simulink model "new_PV_array"  (Simulink 8.5)
settings: Solver=ode45  StartTime=0.0  StopTime=10  RelTol=1e-3
libraries: powerlib x1
settings Model: Creator=farhanm  LastModifiedBy=jiax
settings DebuggingCC: SolverPrmCheckMsg=warning  FcnCallInpInsideContextMsg=UseLocalSettings
settings ConfigurationSet: Description=SimMechanics 2G

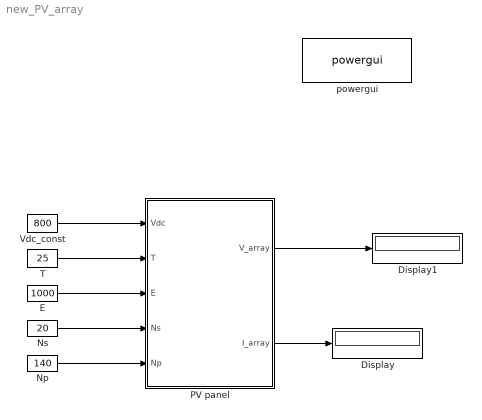
== system new_PV_array ==
  Display : Display
  Display1 : Display
  E : Constant  Value=1000
  Np : Constant  Value=140
  Ns : Constant  Value=20
  "PV panel " : Subsystem  mask{Voc=43.8, Isc=5, Vmpp=35, Impp=4.58, beta_Voc=-0.1, alpha_Isc=0.00002, Ncell=40}
      mask prompts: Voc "Open Circuit Voltage Voc (V)"; Isc "Short Circuit Current Isc (A)"; Vmpp "Voltage at Maximum Power Point Vmpp (V)"; Impp "Current at Maximum Power Point Impp (A)"; beta_Voc "Temperature Coefficient of Voc (%/deg.C)"; alpha_Isc "Temperature Coefficient of Isc (%/deg.C)"; Ncell "Cells per Module (Ncell)"
  T : Constant  Value=25
  Vdc_const : Constant  Value=800
  powergui : powerlib/powergui  Priority=1  SimulationMode=Discrete  SolverType=Tustin/Backward Euler (TBE)  SampleTime=50e-6  frequency=60  SPID=off  DisableSnubberDevices=off  DisableRonSwitches=off  DisableVfSwitches=off  SwTol=0  DisplayEquations=off  Interpol=off  methode=off  Ts=0  FunctionMessages=off  echomessages=off  HookPort=off  EnableUseOfTLC=off  x0status=blocks  frequencyindice=50  Pbase=100e6  ErrMax=1e-4  Iterations=50  UnitsV=kV  UnitsW=MW  buscounter=0  RestoreLinks=warning  ResistiveCurrentMeasurement=off  Frange=[0:2:500]  Ylog=off  Xlog=on  ShowGrid=off  save=off  variable=ZData  structure=0  ZoomFFT=off  StartTime=0.0  cycles=1  DisplayStyle=1  fundamental=60  FreqAxis=off  MaxFrequency=1000  frequencyindicesteady=1  RmsSteady=1  display=off
  wires:
  T/1 -> "PV panel "/2(T)
  E/1 -> "PV panel "/3(E)
  Np/1 -> "PV panel "/5(Np)
  Ns/1 -> "PV panel "/4(Ns)
  "PV panel "/1(V_array) -> Display1/1
  Vdc_const/1 -> "PV panel "/1(Vdc)
  "PV panel "/2(I_array) -> Display/1

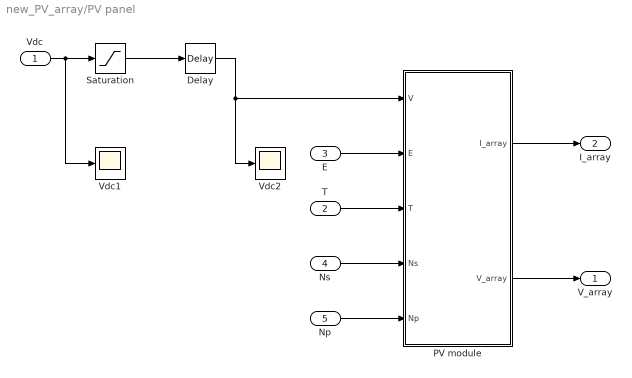
== system new_PV_array/PV panel  ==
  Vdc : Inport
  T : Inport  Port=2
  E : Inport  Port=3
  Ns : Inport  Port=4
  Np : Inport  Port=5
  Delay : TransportDelay  DelayTime=0.05
  PV module : Subsystem
  Saturation : Saturate  UpperLimit=876  LowerLimit=0
  Vdc1 : Scope
      settings: SaveName=ScopeData19
  Vdc2 : Scope
      settings: SaveName=ScopeData20
  V_array : Outport
  I_array : Outport  Port=2
  wires:
  Saturation/1 -> Delay/1
  E/1 -> PV module/2(E)
  T/1 -> PV module/3(T)
  Vdc/1 -> Saturation/1, Vdc1/1
  Delay/1 -> PV module/1(V), Vdc2/1
  Ns/1 -> PV module/4(Ns)
  Np/1 -> PV module/5(Np)
  PV module/1(I_array) -> I_array/1
  PV module/2(V_array) -> V_array/1

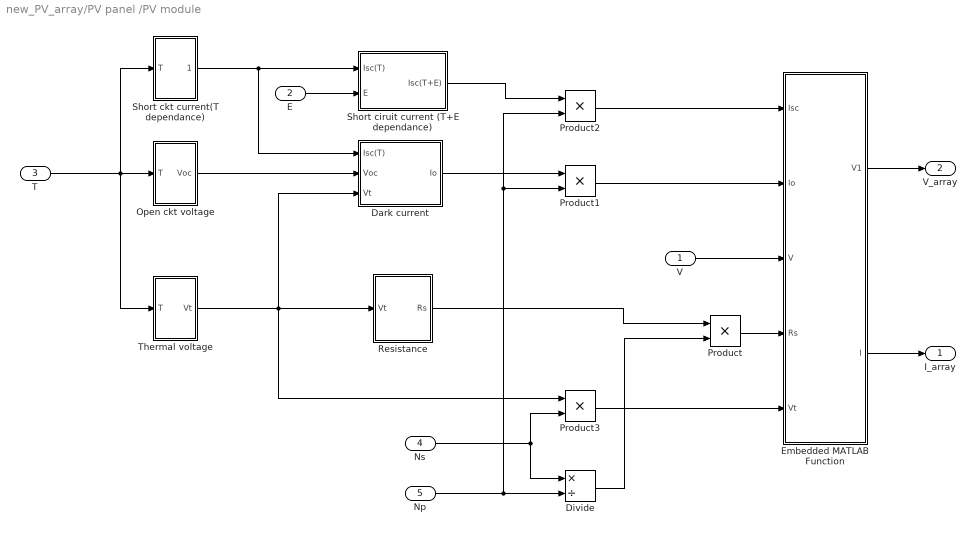
== system new_PV_array/PV panel /PV module ==
  V : Inport
  E : Inport  Port=2
  T : Inport  Port=3
  Ns : Inport  Port=4
  Np : Inport  Port=5
  Dark current : Subsystem
  Divide : Product  Inputs=*/
  Embedded MATLAB Function : MATLAB Function  TreatAsAtomicUnit=on
  Open ckt voltage : Subsystem
  Product{,1..3} (4 alike) : Product
  Resistance : Subsystem
  Short ciruit current (T+E dependance) : Subsystem
  "Short ckt current(T dependance) " : Subsystem
  Thermal voltage : Subsystem
  I_array : Outport
  V_array : Outport  Port=2
  wires:
  Thermal voltage/1(Vt) -> Product3/1, Resistance/1(Vt), Dark current/3(Vt)
  T/1 -> "Short ckt current(T dependance) "/1(T), Thermal voltage/1(T), Open ckt voltage/1(T)
  E/1 -> Short ciruit current (T+E dependance)/2(E)
  Open ckt voltage/1(Voc) -> Dark current/2(Voc)
  Embedded MATLAB Function/2(I) -> I_array/1
  Embedded MATLAB Function/1(V1) -> V_array/1
  V/1 -> Embedded MATLAB Function/3(V)
  Ns/1 -> Product3/2, Divide/1
  Np/1 -> Divide/2, Product1/2, Product2/2
  Product/1 -> Embedded MATLAB Function/4(Rs)
  Product1/1 -> Embedded MATLAB Function/2(Io)
  Product2/1 -> Embedded MATLAB Function/1(Isc)
  Product3/1 -> Embedded MATLAB Function/5(Vt)
  Dark current/1(Io) -> Product1/1
  Resistance/1(Rs) -> Product/1
  Divide/1 -> Product/2
  "Short ckt current(T dependance) "/1(Isc(T)) -> Dark current/1(Isc(T)), Short ciruit current (T+E dependance)/1(Isc(T))
  Short ciruit current (T+E dependance)/1(Isc(T+E)) -> Product2/1

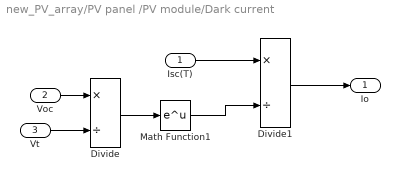
== system new_PV_array/PV panel /PV module/Dark current ==
  Isc(T) : Inport
  Voc : Inport  Port=2
  Vt : Inport  Port=3
  Divide : Product  Inputs=*/
  Divide1 : Product  Inputs=*/
  Math Function1 : Math  SaturateOnIntegerOverflow=on
  Io : Outport
  wires:
  Divide/1 -> Math Function1/1
  Math Function1/1 -> Divide1/2
  Vt/1 -> Divide/2
  Voc/1 -> Divide/1
  Isc(T)/1 -> Divide1/1
  Divide1/1 -> Io/1

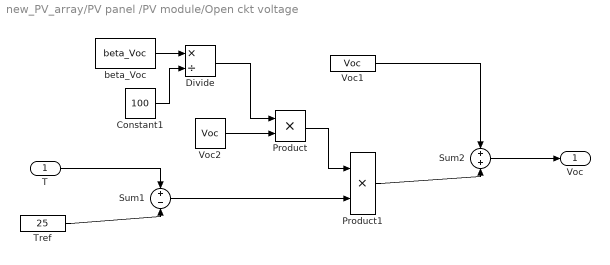
== system new_PV_array/PV panel /PV module/Open ckt voltage ==
  T : Inport
  Constant1 : Constant  Value=100
  Divide : Product  Inputs=*/
  Product : Product
  Product1 : Product  RndMeth=Zero
  Sum1 : Sum  Inputs=+-
  Sum2 : Sum
  Tref : Constant  Value=25
  Voc1 : Constant  Value=Voc
  Voc2 : Constant  Value=Voc
  beta_Voc : Constant  Value=beta_Voc
  Voc : Outport
  wires:
  Tref/1 -> Sum1/2
  T/1 -> Sum1/1
  Sum1/1 -> Product1/2
  Voc1/1 -> Sum2/1
  Product1/1 -> Sum2/2
  Sum2/1 -> Voc/1
  beta_Voc/1 -> Divide/1
  Constant1/1 -> Divide/2
  Divide/1 -> Product/1
  Voc2/1 -> Product/2
  Product/1 -> Product1/1

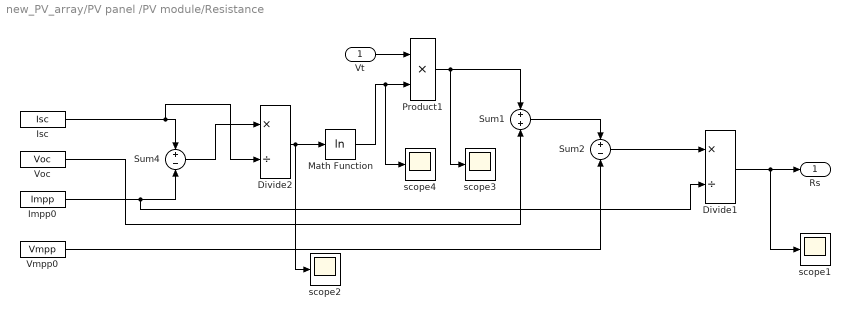
== system new_PV_array/PV panel /PV module/Resistance ==
  Vt : Inport
  Divide1 : Product  Inputs=*/
  Divide2 : Product  Inputs=*/
  Impp0 : Constant  Value=Impp
  Isc : Constant  Value=Isc
  Math Function : Math  Operator=log  SaturateOnIntegerOverflow=on
  Product1 : Product  RndMeth=Zero
  Sum1 : Sum
  Sum2 : Sum  Inputs=+-
  Sum4 : Sum  Inputs=+-
  Vmpp0 : Constant  Value=Vmpp
  Voc : Constant  Value=Voc
  scope{1..4} (4 alike) : Scope
      scope1 settings: SaveName=ScopeData10
      scope2 settings: SaveName=ScopeData11
      scope3 settings: SaveName=ScopeData12
      scope4 settings: SaveName=ScopeData13
  Rs : Outport
  wires:
  Isc/1 -> Sum4/1, Divide2/2
  Impp0/1 -> Sum4/2, Divide1/2
  Divide2/1 -> Math Function/1, scope2/1
  Voc/1 -> Sum1/2
  Product1/1 -> Sum1/1, scope3/1
  Sum1/1 -> Sum2/1
  Vmpp0/1 -> Sum2/2
  Sum2/1 -> Divide1/1
  Divide1/1 -> Rs/1, scope1/1
  Vt/1 -> Product1/1
  Sum4/1 -> Divide2/1
  Math Function/1 -> Product1/2, scope4/1

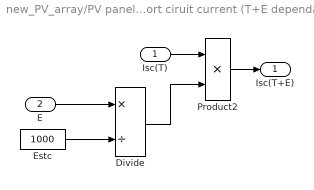
== system new_PV_array/PV panel /PV module/Short ciruit current (T+E dependance) ==
  Isc(T) : Inport
  E : Inport  Port=2
  Divide : Product  Inputs=*/
  Estc : Constant  Value=1000
  Product2 : Product  RndMeth=Zero
  Isc(T+E) : Outport
  wires:
  E/1 -> Divide/1
  Estc/1 -> Divide/2
  Divide/1 -> Product2/2
  Product2/1 -> Isc(T+E)/1
  Isc(T)/1 -> Product2/1

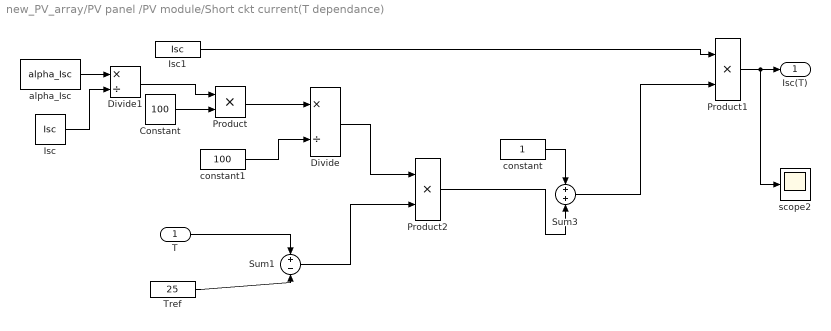
== system new_PV_array/PV panel /PV module/Short ckt current(T dependance)  ==
  T : Inport
  Constant : Constant  Value=100
  Divide : Product  Inputs=*/
  Divide1 : Product  Inputs=*/
  Isc : Constant  Value=Isc
  Isc1 : Constant  Value=Isc
  Product : Product
  Product1 : Product  RndMeth=Zero
  Product2 : Product  RndMeth=Zero
  Sum1 : Sum  Inputs=+-
  Sum3 : Sum
  Tref : Constant  Value=25
  alpha_Isc : Constant  Value=alpha_Isc
  constant : Constant
  constant1 : Constant  Value=100
  scope2 : Scope
      settings: SaveName=ScopeData16
  Isc(T) : Outport
  wires:
  Isc1/1 -> Product1/1
  constant1/1 -> Divide/2
  T/1 -> Sum1/1
  Tref/1 -> Sum1/2
  Product1/1 -> Isc(T)/1, scope2/1
  Divide/1 -> Product2/1
  Sum1/1 -> Product2/2
  constant/1 -> Sum3/1
  Product2/1 -> Sum3/2
  Sum3/1 -> Product1/2
  alpha_Isc/1 -> Divide1/1
  Isc/1 -> Divide1/2
  Divide1/1 -> Product/1
  Constant/1 -> Product/2
  Product/1 -> Divide/1

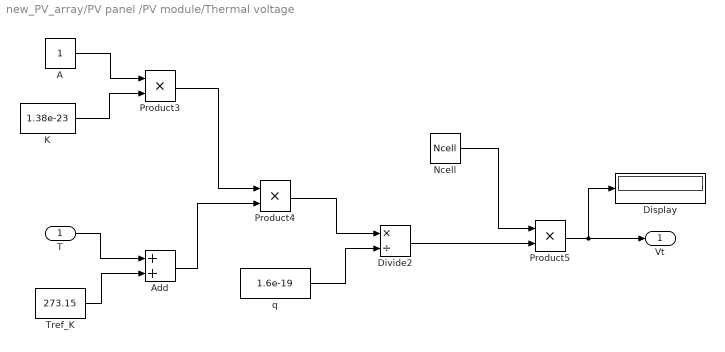
== system new_PV_array/PV panel /PV module/Thermal voltage ==
  T : Inport
  A : Constant
  Add : Sum
  Display : Display
  Divide2 : Product  Inputs=*/
  K : Constant  Value=1.38e-23
  Ncell : Constant  Value=Ncell
  Product3 : Product
  Product4 : Product
  Product5 : Product
  Tref_K : Constant  Value=273.15
  q : Constant  Value=1.6e-19
  Vt : Outport
  wires:
  T/1 -> Add/1
  Tref_K/1 -> Add/2
  A/1 -> Product3/1
  K/1 -> Product3/2
  Product3/1 -> Product4/1
  Add/1 -> Product4/2
  Product4/1 -> Divide2/1
  q/1 -> Divide2/2
  Product5/1 -> Display/1, Vt/1
  Ncell/1 -> Product5/1
  Divide2/1 -> Product5/2

== matlab function PV panel /PV module/Embedded MATLAB Function ==
  data: Isc input double; V1 output double; Io input double; I output double; V input double; Rs input double; Vt input double
function [V1,I] = fcn(Isc, Io,V,Rs,Vt)
 
 %% Newton Raphson Method used in power factory
Istart=0.01;
FI0=0; 
FpI0=0; 
I1=Istart; 

FI1=0; 
FpI1=0; 
I2=I1; 

FI2=0; 
FpI2=0; 
I3=I2; 

FI3=0; 
FpI3=0; 
I4=4.58;
 
 
FI0=Istart-Isc+Io*(exp((V+Istart*Rs)/Vt)-1);
FpI0=1+Io*(exp((V+Istart*Rs)/Vt))*Rs/Vt;
I1=Istart-FI0/FpI0;

FI1=I1-Isc+Io*(exp((V+I1*Rs)/Vt)-1);
FpI1=1+Io*(exp((V+I1*Rs)/Vt))*Rs/Vt;
I2=I1-FI1/FpI1;

FI2=I2-Isc+Io*(exp((V+I2*Rs)/Vt)-1);
FpI2=1+Io*(exp((V+I2*Rs)/Vt))*Rs/Vt;
I3=I2-FI2/FpI2;

FI3=I3-Isc+Io*(exp((V+I3*Rs)/Vt)-1);
FpI3=1+Io*(exp((V+I3*Rs)/Vt))*Rs/Vt;
I4=I3-FI3/FpI3;
I=I4
V1=V;
